simulink model "nonlinear_dynamics"  (R2024b)
settings: Solver=VariableStepAuto  StartTime=0.0  StopTime=10.0  RelTol=1e-3
undefined symbols (not defined in the file): config
settings Model: Creator=kaleb  LastModifiedBy=kaleb
settings DataIOCC: ExternalInput=getinputstruct(op_trim1)  InitialState=getstatestruct(op_trim1)  LoadExternalInput=on  LoadInitialState=on

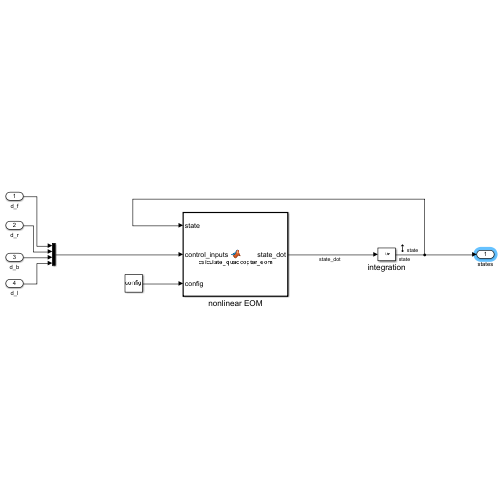
[thumbnail: Simulink's stored preview of the top-level diagram]
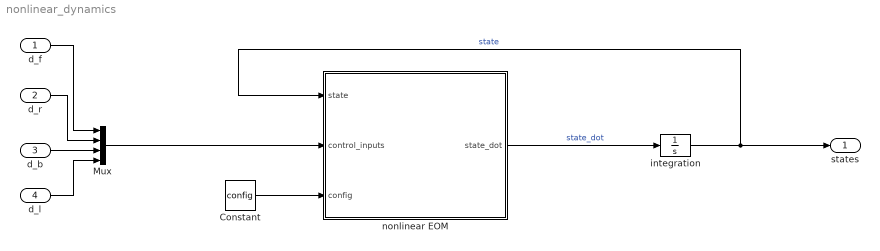
== system nonlinear_dynamics ==
  d_f : Inport
  d_r : Inport  Port=2
  d_b : Inport  Port=3
  d_l : Inport  Port=4
  Constant : Constant  Value=config
  Mux : Mux
  integration : Integrator  InitialCondition=[0,0,0 ,0,0,0 ,0,0,0 ,0,0,0]'
  nonlinear EOM : MATLAB Function  TreatAsAtomicUnit=on
  states : Outport
  wires:
  nonlinear EOM/1(state_dot) -> integration/1  "state_dot"
  Constant/1 -> nonlinear EOM/3(config)
  d_f/1 -> Mux/1
  d_r/1 -> Mux/2
  d_b/1 -> Mux/3
  d_l/1 -> Mux/4
  Mux/1 -> nonlinear EOM/2(control_inputs)
  integration/1 -> states/1, nonlinear EOM/1(state)  "state"

== matlab function nonlinear_dynamics/nonlinear EOM ==
  data: state input; control_inputs input; config input; state_dot output
%% Equation of motion calculation
function state_dot = calculate_quadcopter_eom(state, control_inputs, config)

l_f = config(1);
l_r = config(2);
l_b = config(3);
l_l = config(4);

% state_dot = zeros(12, 1);

t_motor = 31/1000;   % Motor thickness (m)
t_prop = 2/1000;    % Propeller thickness (m)
d_cube = 0.10;    % Cube dimension (m)
m_motor = 58/1000;   % Motor mass (kg)
m_prop = 21/1000;    % Propeller mass (kg)
m_arm = 65/1000;     % Arm mass (kg)
m_cube = 0.69;    % Cube mass (kg)
r_motor = 28/1000;   % Motor radius (m)
r_prop = 25.4/100;    % Propeller radius (m)

g = 9.81; % Gravity (kg/m^2)
k1 = 1;   % Thrust coefficient
k2 = 0.2; % Torque coefficient

[CG_matrix, J_matrix_body, m_tot] = calculate_CG_Moment_of_inertia(config);

X_cg = CG_matrix(1);
Y_cg = CG_matrix(2);

% Function to calculate the equations of motion of the quadcopter
% Inputs:
%   state: [pn; pe; h; u; v; w; phi; theta; psi; p; q; r]
%   control_inputs: [delta_f; delta_r; delta_b; delta_l]
%   J_matrix_body: Moment of inertia matrix [Jx, Jy, Jz]
%   m_tot: Total mass of the quadcopter
%   k1: Thrust coefficient
%   k2: Torque coefficient
%   g: Gravitational acceleration
%   l_f, l_r, l_b, l_l: Individual arm lengths for front, right, back, and left rotors
% Outputs:
%   state_dot: Time derivatives of the state vector
% load_constant_values

% Extract state variables
pn = state(1); pe = state(2); h = state(3);
u = state(4); v = state(5); w = state(6);
phi = state(7); theta = state(8); psi = state(9);
p = state(10); q = state(11); r = state(12);
% 
% Extract control inputs
delta_f = control_inputs(1);
delta_r = control_inputs(2);
delta_b = control_inputs(3);
delta_l = control_inputs(4);

% Position Dynamics
position_matrix = [
    cos(theta)*cos(psi), sin(phi)*sin(theta)*cos(psi) - cos(phi)*sin(psi), cos(phi)*sin(theta)*cos(psi) + sin(phi)*sin(psi);
    cos(theta)*sin(psi), sin(phi)*sin(theta)*sin(psi) + cos(phi)*cos(psi), cos(phi)*sin(theta)*sin(psi) - sin(phi)*cos(psi);
    sin(theta), -sin(phi)*cos(theta), -cos(phi)*cos(theta)
    ];
position_vector = [u; v; w];
position_dot = position_matrix * position_vector;

% Linear Velocity Dynamics
linear_velocity_matrix = [
    0, r, -q;
    -r, 0, p;
    q, -p, 0
    ];
gravity_vector = [-g*sin(theta); g*cos(theta)*sin(phi); g*cos(theta)*cos(phi)];
control_force = [0; 0; -k1 * (delta_f + delta_r + delta_b + delta_l) / m_tot];
linear_velocity_dot = linear_velocity_matrix * [u; v; w] + gravity_vector + control_force;

% Angular Velocity Dynamics
angular_velocity_matrix = [
    1, sin(phi)*tan(theta), cos(phi)*tan(theta);
    0, cos(phi), -sin(phi);
    0, sin(phi)/cos(theta), cos(phi)/cos(theta)
    ];
angular_velocity_dot = angular_velocity_matrix * [p; q; r];

% Rotational Dynamics
% Torques due to rotor thrusts
tau_x = - (l_r-Y_cg) * k1 * delta_r - (l_l-Y_cg) * k1 * delta_l; % Front-back torques
tau_y = (l_f-X_cg) * k1 * delta_f + (l_b-X_cg) * k1 * delta_b; % Right-left torques
tau_z = k2 * (-delta_f + delta_r - delta_b + delta_l); % Yaw torque due to rotor drag

% Total torques
control_torque = [tau_x; tau_y; tau_z];

% Gyroscopic effects
rotational_dynamics_matrix = [
    (J_matrix_body(2, 2) - J_matrix_body(3, 3)) / J_matrix_body(1, 1), 0, 0;
    0, (J_matrix_body(3, 3) - J_matrix_body(1, 1)) / J_matrix_body(2, 2), 0;
    0, 0, (J_matrix_body(1, 1) - J_matrix_body(2, 2)) / J_matrix_body(3, 3)
    ];
rotational_coupling = [q * r; p * r; p * q];
rotational_velocity_dot = rotational_dynamics_matrix * rotational_coupling + (J_matrix_body \ control_torque);
rotational_velocity_dot = inv(J_matrix_body) * (control_torque - cross([p;q;r], J_matrix_body*[p;q;r]));


% Combine EOMs
state_dot = [position_dot; linear_velocity_dot; angular_velocity_dot; rotational_velocity_dot];
end
